simulink model "botsmosfet"  (R2014a)
settings: Solver=ode15s  StartTime=0.0  StopTime=1  RelTol=1e-3
libraries: fl_lib x11, nesl_utility x4, elec_lib x3
settings Model: Creator=laca  LastModifiedBy=laca

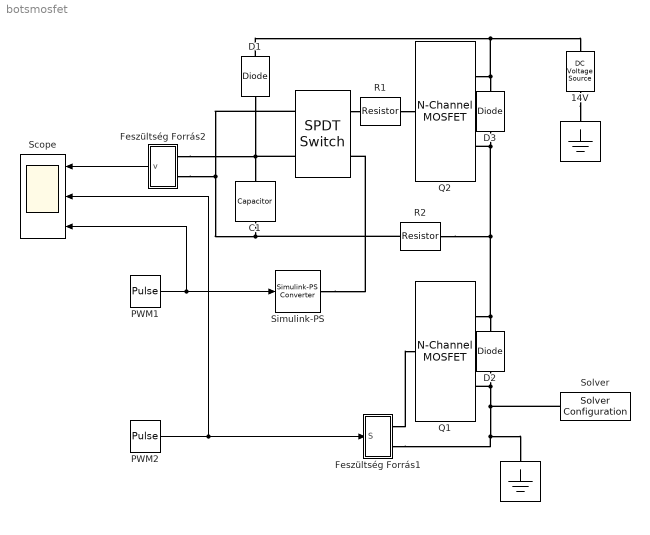
== system botsmosfet ==
  " " : fl_lib/Electrical/Electrical Elements/Electrical Reference
  "  " : elec_lib/Passive Devices/Switches/SPDT Switch  R_closed=0.01 Ohm  G_open=1e-6 S  Threshold=0 V  model_dynamics=0  t_on=0.001 s  t_off=0.001 s  initial_vT=0 V
  " " : fl_lib/Electrical/Electrical Elements/Electrical Reference
  14V : fl_lib/Electrical/Electrical Sources/DC Voltage Source  v0=12 V
  C1 : fl_lib/Electrical/Electrical Elements/Capacitor  c=1 uF  r=1e-06 Ohm  g=0 1/Ohm  i_specify=off  i_priority=High  i=0 A  v_specify=off  v_priority=High  v=0 V  vc_specify=on  vc_priority=High  vc=0 V
  D1 : fl_lib/Electrical/Electrical Elements/Diode  Vf=0.6 V  Ron=0.01 Ohm  Goff=1e-08 1/Ohm  i_specify=off  i_priority=High  i=0 A  v_specify=off  v_priority=High  v=0 V
  D2 : fl_lib/Electrical/Electrical Elements/Diode  Vf=0.6 V  Ron=0.3 Ohm  Goff=1e-8 1/Ohm  i_specify=off  i_priority=High  i=0 A  v_specify=off  v_priority=High  v=0 V
  D3 : fl_lib/Electrical/Electrical Elements/Diode  Vf=0.6 V  Ron=0.3 Ohm  Goff=1e-8 1/Ohm  i_specify=off  i_priority=High  i=0 A  v_specify=off  v_priority=High  v=0 V
  "Feszültség Forrás1 " : Subsystem
      settings: CopyFcn=set_param(gcb,'LinkStatus','none')
  Feszültség Forrás2 : Subsystem
      settings: CopyFcn=set_param(gcb,'LinkStatus','none')
  PWM1 : DiscretePulseGenerator  PulseType=Time based  Amplitude=10  Period=14*10^-4  PulseWidth=45
  PWM2 : DiscretePulseGenerator  PulseType=Time based  Amplitude=10  Period=14*10^-4  PulseWidth=0.5
  Q1 : elec_lib/Semiconductor Devices/N-Channel MOSFET  parameterization=1  prmDatasheet=1  prmEquCoeff=1  Beta=5 A/V^2  Rds=0.025 Ohm  Id=6 A  Vgs=10 V  Vth=1.7 V  lam=0 1/V  Tmeas=25 C  RS=1e-4 Ohm  RD=0.01 Ohm  C_param=1  C_GS=270 pF  C_GD=80 pF  C_iss=350 pF  C_rss=80 pF  C_oss=0 pF  charge_linearity_param=1  C_OX=200 pF  V_C_OX=-0.5 V  dVth_dT=-6 mV/K  Rds_T2=0.037 Ohm  Tmeas2=125 C  BEXDatasheet=-1.5  BEXEquCoeff=-1.5  TdeviceDatasheet=25 C  TdeviceEquCoeff=25 C  Rth=[ 0 10 ] K/W  thermal_mass_parameterization=1  thermal_mass=[ 0 1 ] J/K  thermal_time_constant=[ 0 10 ] s  thermal_mass_initial_temperatures=[ 25 25 ] C
  Q2 : elec_lib/Semiconductor Devices/N-Channel MOSFET  parameterization=1  prmDatasheet=1  prmEquCoeff=1  Beta=5 A/V^2  Rds=0.025 Ohm  Id=6 A  Vgs=10 V  Vth=1.7 V  lam=0 1/V  Tmeas=25 C  RS=1e-4 Ohm  RD=0.01 Ohm  C_param=1  C_GS=270 pF  C_GD=80 pF  C_iss=350 pF  C_rss=80 pF  C_oss=0 pF  charge_linearity_param=1  C_OX=200 pF  V_C_OX=-0.5 V  dVth_dT=-6 mV/K  Rds_T2=0.037 Ohm  Tmeas2=125 C  BEXDatasheet=-1.5  BEXEquCoeff=-1.5  TdeviceDatasheet=25 C  TdeviceEquCoeff=25 C  Rth=[ 0 10 ] K/W  thermal_mass_parameterization=1  thermal_mass=[ 0 1 ] J/K  thermal_time_constant=[ 0 10 ] s  thermal_mass_initial_temperatures=[ 25 25 ] C
  R1 : fl_lib/Electrical/Electrical Elements/Resistor  R=200 Ohm  i_specify=off  i_priority=High  i=0 A  v_specify=off  v_priority=High  v=0 V
  R2 : fl_lib/Electrical/Electrical Elements/Resistor  R=200 Ohm  i_specify=off  i_priority=High  i=0 A  v_specify=off  v_priority=High  v=0 V
  Scope : Scope  NumInputPorts=3
      settings: YMin=0~-13~-5  YMax=11.5~0~5
  "Simulink-PS " : nesl_utility/Simulink-PS Converter  PhysicalDomain=network_engine_domain  SubClassName=ps_input  LeftPortType=input  RightPortType=output  PseudoPeriodic=off  Frequencies=[]  NoiseDistribution=none  NoiseParameters=[]  Unit=V  AffineConversion=off  InputFiltering=off  SimscapeFilterOrder=1  InputFilterTimeConstant=.001  UdotUserProvided=0
  Solver : nesl_utility/Solver Configuration  PhysicalDomain=network_engine_domain  SubClassName=solver  LeftPortType=input  RightPortType=generic  Accelerate=off  Tones=[]  Harmonics=[]  SimulateNoise=off  Profile=off  UseLocalSampling=off  EnableSwitchedLinearOptims=on  FrequencyDomain=off  UseCCode=off  RelTol=0.001  AbsTol=1e-06  MinStep=1e-09  ToWorkspace=off  DoDC=off  ResidualTolerance=1e-10  UseLocalSolver=off  LocalSolverChoice=NE_BACKWARD_EULER_ADVANCER  LocalSolverSampleTime=.001  DoFixedCost=off  MaxNonlinIter=4  MaxModeIter=4  LinearAlgebra=Sparse  DelaysMemoryBudget=1024  AutomaticFiltering=on  FilteringTimeConstant=0.000001
  wires:
  PWM2/1 -> "Feszültség Forrás1 "/1(S), Scope/2
  Feszültség Forrás2/1(v) -> Scope/1
  PWM1/1 -> Scope/3, "Simulink-PS "/1
  connections:
  Q2/RConn1 -- 14V/LConn1 -- D1/LConn1 -- D3/RConn1
  D1/RConn1 -- Feszültség Forrás2/LConn1 -- "  "/RConn1 -- C1/LConn1
  D2/RConn1 -- R2/LConn1 -- D3/LConn1 -- Q2/RConn2 -- Q1/RConn1
  14V/RConn1 -- " "/LConn1
  Q1/RConn2 -- Solver/RConn1 -- "Feszültség Forrás1 "/RConn2 -- " "/LConn1 -- D2/LConn1
  "  "/LConn2 -- R1/RConn1
  R1/LConn1 -- Q2/LConn1
  "Simulink-PS "/RConn1 -- "  "/LConn1
  "Feszültség Forrás1 "/RConn1 -- Q1/LConn1
  Feszültség Forrás2/LConn2 -- "  "/RConn2 -- R2/RConn1 -- C1/RConn1

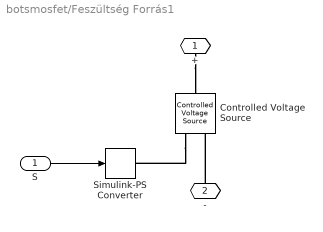
== system botsmosfet/Feszültség Forrás1  ==
  S : Inport
  Controlled Voltage Source : fl_lib/Electrical/Electrical Sources/Controlled Voltage Source
  Simulink-PS Converter : nesl_utility/Simulink-PS Converter  PhysicalDomain=network_engine_domain  SubClassName=ps_input  LeftPortType=input  RightPortType=output  PseudoPeriodic=off  Frequencies=[]  NoiseDistribution=none  NoiseParameters=[]  Unit=V  AffineConversion=off  InputFiltering=off  SimscapeFilterOrder=1  InputFilterTimeConstant=.001  UdotUserProvided=0
  + : PMIOPort  Port=1  Side=Right
  - : PMIOPort  Port=2  Side=Right
  wires:
  S/1 -> Simulink-PS Converter/1
  connections:
  +/RConn1 -- Controlled Voltage Source/LConn1
  -/RConn1 -- Controlled Voltage Source/RConn2
  Controlled Voltage Source/RConn1 -- Simulink-PS Converter/RConn1

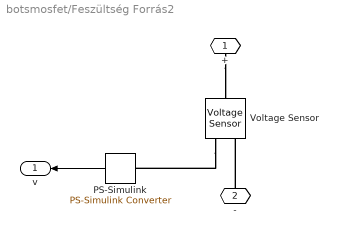
== system botsmosfet/Feszültség Forrás2 ==
  PS-Simulink : nesl_utility/PS-Simulink Converter  PhysicalDomain=network_engine_domain  SubClassName=ps_output  LeftPortType=input  RightPortType=output  PseudoPeriodic=off  Frequencies=[]  Unit=V  AffineConversion=off
  Voltage Sensor : fl_lib/Electrical/Electrical Sensors/Voltage Sensor
  + : PMIOPort  Port=1  Side=Left
  - : PMIOPort  Port=2  Side=Left
  v : Outport
  wires:
  PS-Simulink/1 -> v/1
  connections:
  -/RConn1 -- Voltage Sensor/RConn2
  +/RConn1 -- Voltage Sensor/LConn1
  Voltage Sensor/RConn1 -- PS-Simulink/LConn1
